simulink model "sheji_2tu"  (R2020b)
settings: Solver=VariableStepAuto  StartTime=0.0  StopTime=10  RelTol=1e-3
values from neighbouring files (symbols this model uses):
  A = [ 0 1 0 ... (first row only)    [Bujiao_ZuoYe2.m]    (also in fenxi_2.m = [-4 1 0 0 0 0; sheji_1.m = [-1 0 0 0; sheji_1Kong.m = [-1 0 0 0;2 -3 0 0;0 0 2 0;4 -1 2 -4]; sheji_2.m = [-1 0 0 0)
  B = [0 ... (first row only)    [Bujiao_ZuoYe2.m]    (also in fenxi_2.m = [1 3; sheji_1.m = [0;0;1;2]; sheji_1Kong.m = [0;0;1;2]; sheji_2.m = [0;0;1;2])
  C = [0 0 1]    [Bujiao_ZuoYe2.m]    (also in fenxi_2.m = [3 1 0 5 0 0; sheji_1.m = [3 0 1 0]; sheji_1Kong.m = [3 0 1 0]; sheji_2.m = [3 0 1 0])
  D = [0]    [Bujiao_ZuoYe2.m]    (also in sheji_1.m = zeros(1,1); sheji_2.m = zeros(1,1); sheji_3.m)
  G = T*[0;0;G_]    [sheji_2.m]    (also in sheji_3.m; sheji_3Kong.m = T*G2)
  Init = [-0.1 0.1 0.2 -0.3]    [sheji_1.m]    (also in sheji_2.m = [-0.1 0.1 0.2 0.22]; sheji_3.m = [-0.1 0.1 0.2 -0.05]; sheji_3Kong.m)
settings Model: Creator=19017  LastModifiedBy=19017

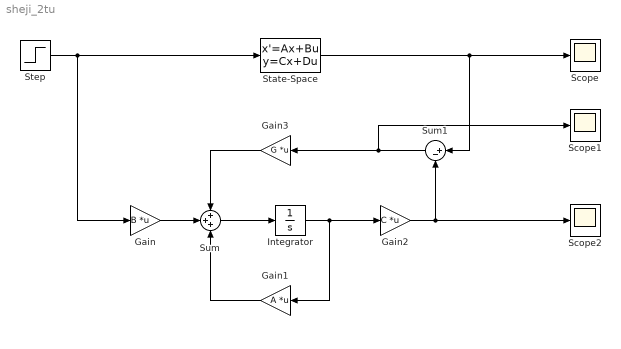
== system sheji_2tu ==
  Gain : Gain  Gain=B  Multiplication=Matrix(K*u)
  Gain1 : Gain  Gain=A  Multiplication=Matrix(K*u)
  Gain2 : Gain  Gain=C  Multiplication=Matrix(K*u)
  Gain3 : Gain  Gain=G  Multiplication=Matrix(K*u)
  Integrator : Integrator
  Scope : Scope
  Scope1 : Scope
  Scope2 : Scope
  State-Space : StateSpace  A=A  B=B  C=C  D=D  InitialCondition=Init
  Step : Step  SampleTime=0
  Sum : Sum  Inputs=+++
  Sum1 : Sum  Inputs=|+-
  wires:
  Step/1 -> Gain/1, State-Space/1
  State-Space/1 -> Sum1/1, Scope/1
  Integrator/1 -> Gain1/1, Gain2/1
  Sum/1 -> Integrator/1
  Gain2/1 -> Scope2/1, Sum1/2
  Gain/1 -> Sum/2
  Gain1/1 -> Sum/3
  Sum1/1 -> Scope1/1, Gain3/1
  Gain3/1 -> Sum/1
